simulink model "send_command_xplane_9"  (R2016a)
settings: Solver=VariableStepAuto  StartTime=0.0  StopTime=inf  RelTol=1e-3
libraries: etargetslib x1, dspnetwork x1
settings Model: Creator=iwin  LastModifiedBy=iwin

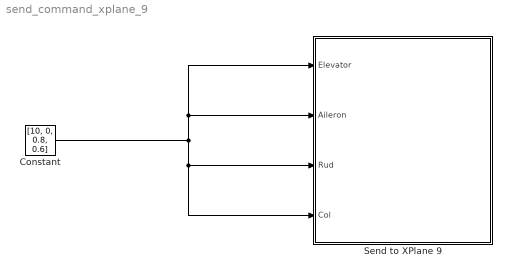
== system send_command_xplane_9 ==
  Constant : Constant  Value=[10, 0, 0.8, 0.6]  OutDataTypeStr=single
  Send to XPlane 9 : Subsystem  Description=|  mask(Send Commands to X-Plane 10){remoteURL='127.0.0.1', remotePort=49000}
      | Done by: Mohamed Abdelkader
      | Contact for updates: mohamedashraf123@gmail.com
      mask prompts: remoteURL "Remote IP address (default='127.0.0.1'): X-Plane 9 IP"; remotePort "Remote IP port:X-Plane 9 port(default=49000)"
      mask help:
      | Sends Control Surfaces Commands to Xplane10
      | Throttle in [0,1]
      | Elevator, Ailerons, rudder, nosewheel in [-1,1]
      mask TypeOptions remoteURL: UDP Send/remoteURL
  wires:
  Constant/1 -> Send to XPlane 9/4(Col), Send to XPlane 9/3(Rud), Send to XPlane 9/1(Elevator), Send to XPlane 9/2(Aileron)

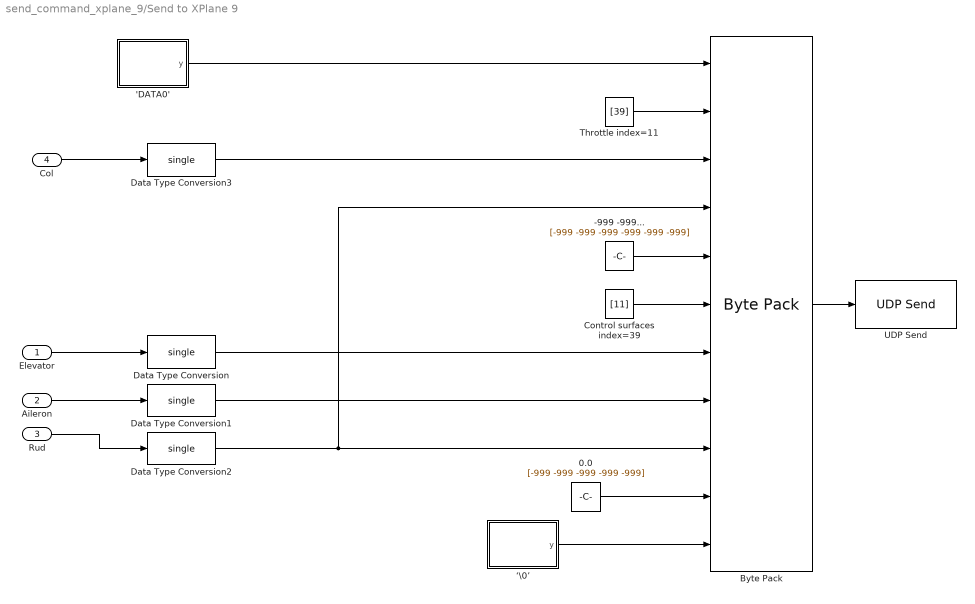
== system send_command_xplane_9/Send to XPlane 9 ==
  Elevator : Inport
  Aileron : Inport  Port=2
  Rud : Inport  Port=3
  Col : Inport  Port=4
  'DATA0' : MATLAB Function  TreatAsAtomicUnit=on
  -999 -999... : Constant  Value=[-999 -999 -999 -999 -999 -999]  OutDataTypeStr=int32  SampleTime=-1
  0.0 : Constant  Value=[-999 -999 -999 -999 -999]  OutDataTypeStr=int32  SampleTime=-1
  Byte Pack : etargetslib/Byte Pack  datatypes={'uint8','uint32','single','single','int32','uint32','single','single','single', 'int32', 'uint8'}  byteAlign=1
  Control surfaces index=39 : Constant  Value=[11]  OutDataTypeStr=uint32  SampleTime=-1
  Data Type Conversion : DataTypeConversion  OutMin=[0]  OutMax=[1.0]  OutDataTypeStr=single
  Data Type Conversion1 : DataTypeConversion  OutMin=[-1.0]  OutMax=[1.0]  OutDataTypeStr=single
  Data Type Conversion2 : DataTypeConversion  OutMin=[-1.0]  OutMax=[1.0]  OutDataTypeStr=single
  Data Type Conversion3 : DataTypeConversion  OutMin=[-1.0]  OutMax=[1.0]  OutDataTypeStr=single
  Throttle index=11 : Constant  Value=[39]  OutDataTypeStr=uint32  SampleTime=-1
  UDP Send : dspnetwork/UDP Send  remoteURL=remoteURL  remotePort=49000  localURL='0.0.0.0'  localPortSource=Automatically determine  localPort=-1  sampletime=-1  separateLengthPort=0
  ‘\0’ : MATLAB Function  TreatAsAtomicUnit=on
  wires:
  Aileron/1 -> Data Type Conversion1/1
  Byte Pack/1 -> UDP Send/1
  Throttle index=11/1 -> Byte Pack/2
  'DATA0'/1(y) -> Byte Pack/1
  Elevator/1 -> Data Type Conversion/1
  Rud/1 -> Data Type Conversion2/1
  Col/1 -> Data Type Conversion3/1
  ‘\0’/1(y) -> Byte Pack/11
  Data Type Conversion3/1 -> Byte Pack/3
  -999 -999.../1 -> Byte Pack/5
  0.0/1 -> Byte Pack/10
  Control surfaces index=39/1 -> Byte Pack/6
  Data Type Conversion/1 -> Byte Pack/7
  Data Type Conversion1/1 -> Byte Pack/8
  Data Type Conversion2/1 -> Byte Pack/4, Byte Pack/9

== matlab function send_command_xplane_9/Send to XPlane 9/'DATA0' ==
  data: y output
function y = fcn()
%#codegen
%y=uint8(zeros(1,77));
y = uint8('DATA0');

== matlab function send_command_xplane_9/Send to XPlane 9/‘\0’ ==
  data: y output
function y = fcn()
%#codegen
%y=uint8(zeros(1,77));
y = uint8('\0');
